simulink model "Zadatak3"  (R2013b)
settings: Solver=ode45  StartTime=0.0  StopTime=50  RelTol=1e-3
settings Model: Creator=Korisnik  LastModifiedBy=Korisnik

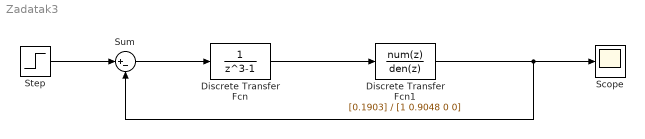
== system Zadatak3 ==
  Discrete Transfer Fcn : DiscreteTransferFcn  Denominator=[1 0 0 -1]  SampleTime=1
  Discrete Transfer Fcn1 : DiscreteTransferFcn  Numerator=[0.1903]  Denominator=[1 0.9048 0 0]
  Scope : Scope
      settings: TimeRange=50  YMin=0  YMax=0.7000000000000001
  Step : Step  SampleTime=0
  Sum : Sum  Inputs=|+-
  wires:
  Step/1 -> Sum/1
  Sum/1 -> Discrete Transfer Fcn/1
  Discrete Transfer Fcn/1 -> Discrete Transfer Fcn1/1
  Discrete Transfer Fcn1/1 -> Sum/2, Scope/1
